simulink model "rst_diagram"  (R2018b)
settings: Solver=VariableStepAuto  StartTime=0.0  StopTime=40  RelTol=1e-3
values from neighbouring files (symbols this model uses):
  den = [10 1]    [cod_teste_RST_1.m]    (also in cod_teste_RST_2.m = [0.1 1.1 1])
  num = 1    [cod_teste_RST_1.m]    (also in cod_teste_RST_2.m)
  R = X(1)    [cod_teste_RST_1.m]    (also in cod_teste_RST_2.m = [1 X(1)])
  S = X(2:end)    [cod_teste_RST_1.m]    (also in cod_teste_RST_2.m = [X(3) X(2)])
  T = sum(PMF)/sum(B)    [cod_teste_RST_1.m]    (also in cod_teste_RST_2.m = sum(Am)/sum(B))
libraries: peAlternativeControllers x1
settings Model: Creator=Carlos Henrique  LastModifiedBy=tarci

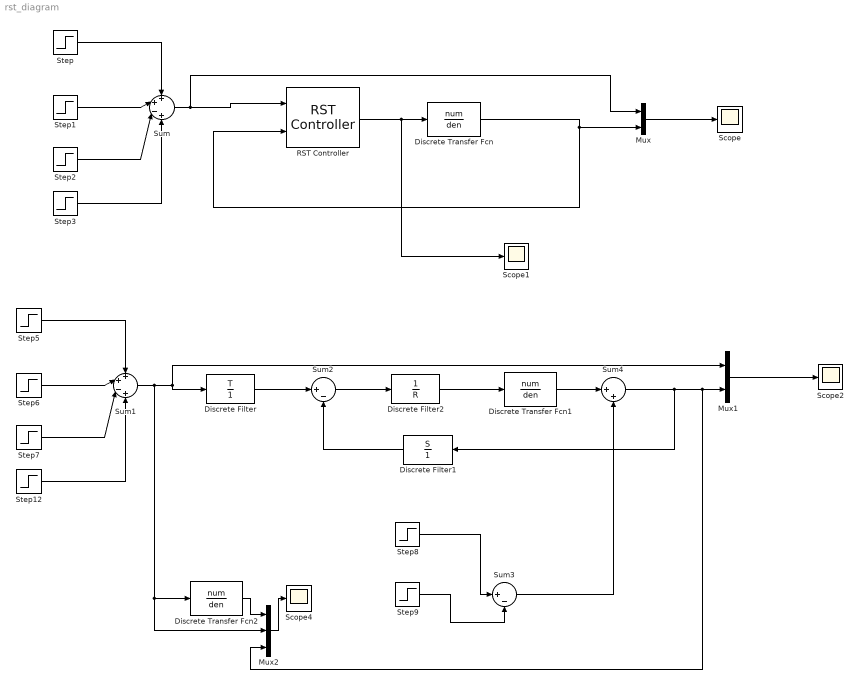
== system rst_diagram ==
  Discrete Transfer Fcn : DiscreteTransferFcn  Numerator=num  Denominator=den
  Discrete Transfer Fcn1 : DiscreteTransferFcn  Numerator=num  Denominator=den
  Discrete Transfer Fcn2 : DiscreteTransferFcn  Numerator=num  Denominator=den
  Discrete Filter : DiscreteFilter  Numerator=T  Denominator=1
  Discrete Filter1 : DiscreteFilter  Numerator=S  Denominator=1
  Discrete Filter2 : DiscreteFilter  Numerator=1  Denominator=R
  Mux : Mux  Inputs=2
  Mux1 : Mux  Inputs=2
  Mux2 : Mux  Inputs=3
  RST Controller : peAlternativeControllers/RST Controller  CtrlParam=Controller polynomials  R=R  S=S  T=T  B=1  A=[1 0.5]  N=5  lam=0.5  d=2  Ts=0.1
  Scope{,1..2,4} (4 alike) : Scope
  Step : Step  Time=0  SampleTime=0
  Step1 : Step  Time=10  After=3  SampleTime=0
  Step12 : Step  Time=30  SampleTime=0
  Step2 : Step  Time=20  After=2  SampleTime=0
  Step3 : Step  Time=30  SampleTime=0
  Step5 : Step  Time=0  SampleTime=0
  Step6 : Step  Time=10  After=3  SampleTime=0
  Step7 : Step  Time=20  After=2  SampleTime=0
  Step8 : Step  Time=10  After=0.3  SampleTime=0
  Step9 : Step  Time=15  After=0.3  SampleTime=0
  Sum : Sum  Inputs=++-+
  Sum1 : Sum  Inputs=++-+
  Sum2 : Sum  Inputs=|+-
  Sum3 : Sum  Inputs=|+-
  Sum4 : Sum  Inputs=|++
  wires:
  RST Controller/1 -> Scope1/1, Discrete Transfer Fcn/1
  Discrete Transfer Fcn/1 -> RST Controller/2, Mux/2
  Step2/1 -> Sum/3
  Step1/1 -> Sum/2
  Step/1 -> Sum/1
  Sum/1 -> Mux/1, RST Controller/1
  Mux/1 -> Scope/1
  Step3/1 -> Sum/4
  Discrete Filter/1 -> Sum2/1
  Discrete Filter1/1 -> Sum2/2
  Sum2/1 -> Discrete Filter2/1
  Discrete Filter2/1 -> Discrete Transfer Fcn1/1
  Mux1/1 -> Scope2/1
  Step8/1 -> Sum3/1
  Discrete Transfer Fcn1/1 -> Sum4/1
  Sum4/1 -> Discrete Filter1/1, Mux2/3, Mux1/2
  Step5/1 -> Sum1/1
  Step6/1 -> Sum1/2
  Step7/1 -> Sum1/3
  Step12/1 -> Sum1/4
  Sum1/1 -> Mux2/2, Discrete Transfer Fcn2/1, Discrete Filter/1, Mux1/1
  Discrete Transfer Fcn2/1 -> Mux2/1
  Mux2/1 -> Scope4/1
  Step9/1 -> Sum3/2
  Sum3/1 -> Sum4/2
